simulink model "differential_car"  (R2018a)
settings: Solver=FixedStepDiscrete  StartTime=0.0  StopTime=500  FixedStep=0.1  RelTol=1e-3
values from neighbouring files (symbols this model uses):
  K_omega = 0.000972    [runMain.m]
  Kd = 6    [runMain.m]
  Kp = 1    [runMain.m]
  L = 1    [runMain.m]
  r = 7.3    [runMain.m]
  theta0 = 0    [runMain.m]
  v_0 = 0.3    [runMain.m]
  x0 = 4    [runMain.m]
  y0 = 0    [runMain.m]
undefined symbols (not defined in the file or in its folder): DiscIntNeverNeededParam, evalt2
libraries: simulink x1
settings Model: Creator=Johnhui  LastModifiedBy=Johnhui

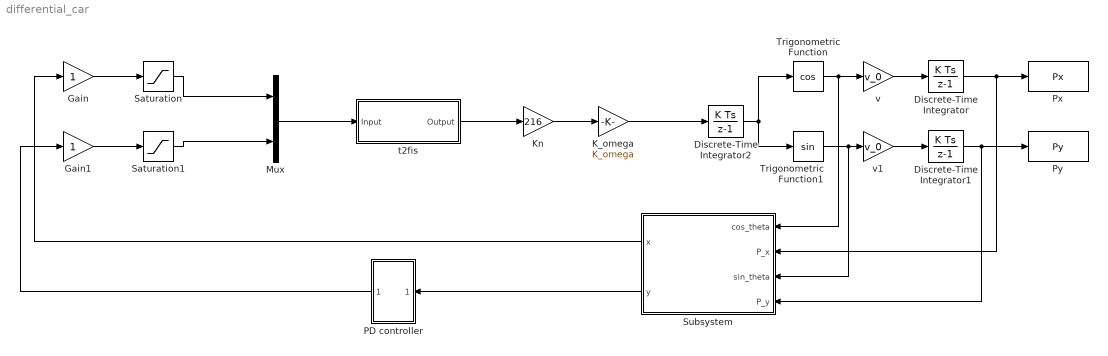
== system differential_car ==
  Discrete-Time Integrator : DiscreteIntegrator  InitialCondition=x0  SampleTime=-1  ICPrevOutput=DiscIntNeverNeededParam  ICPrevScaledInput=DiscIntNeverNeededParam
  Discrete-Time Integrator1 : DiscreteIntegrator  InitialCondition=y0  SampleTime=-1  ICPrevOutput=DiscIntNeverNeededParam  ICPrevScaledInput=DiscIntNeverNeededParam
  Discrete-Time Integrator2 : DiscreteIntegrator  InitialCondition=theta0  SampleTime=-1  ICPrevOutput=DiscIntNeverNeededParam  ICPrevScaledInput=DiscIntNeverNeededParam
  Gain : Gain
  Gain1 : Gain
  K_omega : Gain  Gain=K_omega
  Kn : Gain  Gain=216
  Mux : Mux  Inputs=2
  PD controller : Subsystem
  Px : ToWorkspace  VariableName=Px  SaveFormat=Structure With Time  SampleTime=-1
  Py : ToWorkspace  VariableName=Py  SaveFormat=Structure With Time  SampleTime=-1
  Saturation : Saturate  UpperLimit=2  LowerLimit=-2
  Saturation1 : Saturate  UpperLimit=2  LowerLimit=-2
  Subsystem : Subsystem
  Trigonometric Function : Trigonometry  Operator=cos
  Trigonometric Function1 : Trigonometry
  t2fis : Subsystem  AncestorBlock=Fuzzy_Type2_Lib/Interval Type-2 Fuzzy Logic Controller  mask(Type-2 Fuzzy Logic Controller){t2fisSim=t2fisSim}
      mask prompts: t2fisSim "t2fis name in Workspace or File Name"
      mask Display: image(imread('MemberShipMask.jpg'))
  v : Gain  Gain=v_0
  "v1 " : Gain  Gain=v_0
  wires:
  Kn/1 -> K_omega/1
  K_omega/1 -> Discrete-Time Integrator2/1
  Discrete-Time Integrator2/1 -> Trigonometric Function/1, Trigonometric Function1/1
  Trigonometric Function/1 -> Subsystem/1(cos_theta), v/1
  Trigonometric Function1/1 -> Subsystem/3(sin_theta), "v1 "/1
  v/1 -> Discrete-Time Integrator/1
  Discrete-Time Integrator/1 -> Px/1, Subsystem/2(P_x)
  Discrete-Time Integrator1/1 -> Py/1, Subsystem/4(P_y)
  Gain/1 -> Saturation/1
  Gain1/1 -> Saturation1/1
  Saturation/1 -> Mux/1
  Saturation1/1 -> Mux/2
  "v1 "/1 -> Discrete-Time Integrator1/1
  Mux/1 -> t2fis/1(Input)
  t2fis/1(Output) -> Kn/1
  Subsystem/1(x) -> Gain/1
  Subsystem/2(y) -> PD controller/1(In1)
  PD controller/1(Out1) -> Gain1/1

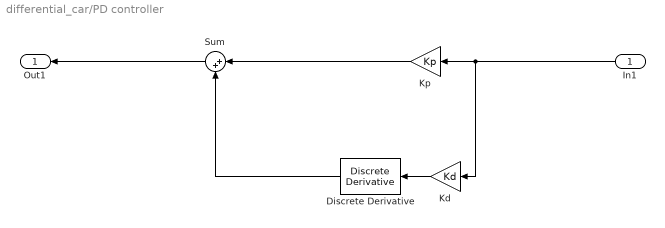
== system differential_car/PD controller ==
  In1 : Inport
  Discrete Derivative : simulink/Discrete/Discrete Derivative  gainval=1.0  ICPrevScaledInput=0.0  OutMin=[]  OutMax=[]  OutDataType=fixdt(1, 16)  OutScaling=2^-10  DoSatur=off
  Kd : Gain  Gain=Kd
  Kp : Gain  Gain=Kp
  Sum : Sum  Inputs=|++
  Out1 : Outport
  wires:
  In1/1 -> Kd/1, Kp/1
  Sum/1 -> Out1/1
  Discrete Derivative/1 -> Sum/2
  Kd/1 -> Discrete Derivative/1
  Kp/1 -> Sum/1

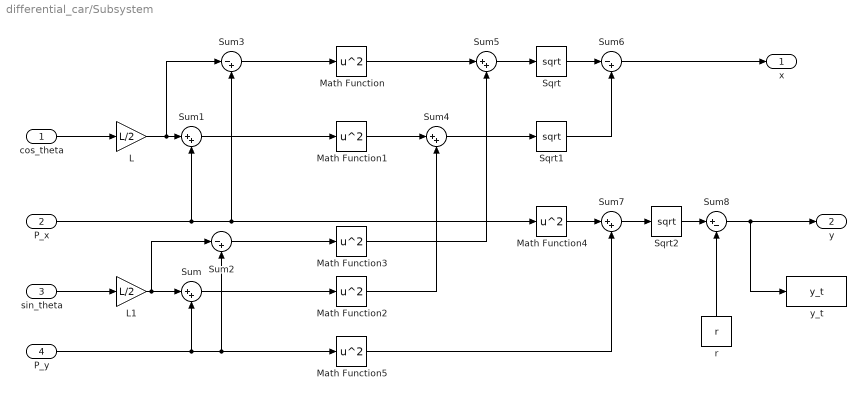
== system differential_car/Subsystem ==
  cos_theta : Inport
  P_x : Inport  Port=2
  sin_theta : Inport  Port=3
  P_y : Inport  Port=4
  L : Gain  Gain=L/2
  L1 : Gain  Gain=L/2
  Math Function{,1..5} (6 alike) : Math  Operator=square  SaturateOnIntegerOverflow=on
  Sqrt : Sqrt  SaturateOnIntegerOverflow=on
  Sqrt1 : Sqrt  SaturateOnIntegerOverflow=on
  Sqrt2 : Sqrt  SaturateOnIntegerOverflow=on
  Sum{,1,4..5,7} (5 alike) : Sum  Inputs=|++
  Sum2 : Sum  Inputs=|-+
  Sum3 : Sum  Inputs=|-+
  Sum6 : Sum  Inputs=|-+
  Sum8 : Sum  Inputs=|+-
  r : Constant  Value=r
  y_t : ToWorkspace  VariableName=y_t  SaveFormat=Structure With Time  SampleTime=-1
  x : Outport
  y : Outport  Port=2
  wires:
  Sum2/1 -> Math Function3/1
  L1/1 -> Sum2/1, Sum/1
  Math Function1/1 -> Sum4/1
  Sqrt2/1 -> Sum8/1
  Sum5/1 -> Sqrt/1
  Math Function2/1 -> Sum4/2
  sin_theta/1 -> L1/1
  L/1 -> Sum3/1, Sum1/1
  Sum8/1 -> y_t/1, y/1
  r/1 -> Sum8/2
  P_y/1 -> Sum2/2, Math Function5/1, Sum/2
  P_x/1 -> Sum3/2, Math Function4/1, Sum1/2
  cos_theta/1 -> L/1
  Math Function3/1 -> Sum5/2
  Sum1/1 -> Math Function1/1
  Math Function/1 -> Sum5/1
  Sum7/1 -> Sqrt2/1
  Sum/1 -> Math Function2/1
  Sum3/1 -> Math Function/1
  Math Function4/1 -> Sum7/1
  Sum4/1 -> Sqrt1/1
  Math Function5/1 -> Sum7/2
  Sqrt/1 -> Sum6/1
  Sum6/1 -> x/1
  Sqrt1/1 -> Sum6/2

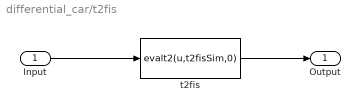
== system differential_car/t2fis ==
  Input : Inport
  t2fis : MATLABFcn  MATLABFcn=evalt2(u,t2fisSim,0)  OutputDimensions=1
  Output : Outport
  wires:
  t2fis/1 -> Output/1
  Input/1 -> t2fis/1
